simulink model "NETWORK"  (Simulink 7.3)
settings: Solver=ode45  StartTime=0.0  StopTime=.6  RelTol=1e-3
undefined symbols (not defined in the file or in its folder): Current, Measurement, Measurements, powerib, q, SampleTime, Syste
libraries: powerlib x9,       x1
settings Model: Creator=me  LastModifiedBy=me  Line=k  SrcBlock="\"(SFunction \""  SrgPort=1  DstFnock=Demux  DstPort=1

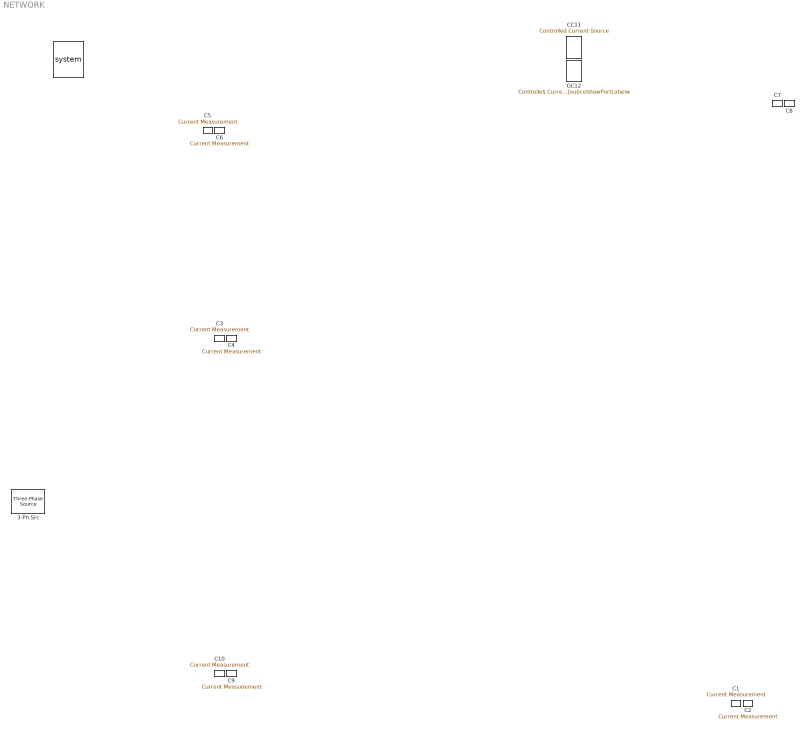
== system NETWORK ==
  3-Ph Src : powerlib/Electrical Sources/Three-Phase Source  DialogController=POWERSYS.PowerSysDialog  SystemSampleTime=-1  Voltage=380  PhaseAngle=0  Frequency=50  InternalConnection=Yn  SpecifyImpedance=on  Resistance=0.8929  Inductance=16.58e-3  ShortCircuitLevel=100e6  BaseVoltage=380  XRratio=7
  C{1..6,10} (7 alike) : powerlib/Measurements/Current Measurement  DialogController=POWERSYS.PowerSysDialog  SystemSampleTime=-1  PhasorSimulation=off  OutputType=Complex  PSBequivalent=0
  C7 : Reference  DialogControllar=POWERSYS.PowerSysDialog  F="ntNam%\t\t      \"Verdana\""  SourceBlocj=powerib/Measurements/Current(Measurement  Currånt="Measurement\""  SystemSampleTime="(  \"-1\""  FunctionWithSeparatEData=off  RTWÍemSecFuncInitTerm=Inherit from`model  RTWMemWecDataParameters="(\"Inherit from model\""  OutputType=Complex  PSBesuivalent="`\u00020\""
      settings: RTWMemSecFuncExecute=|
      | 0"Inherit from model"
      | Š      RTWMemSecDataConstants  "Inherit from model"
  C8 : Refarence  Pgrts="`    [0, 3, 0, 0, 0, q, 1]"  $="BlockRotatkon\t      270"  Di="`logController\t      \"POWMRSYS.PowerSys@ialog\""  SourceBlock=powerlib/Measurements/Current Measurement  SystemSampleTime=-1  PhasorSimulation=off  OutputType=Complex  PSBequivalent=0
  C9 :        DialogController=POWERSYS.PowerSysDialog  ShowPortLabelS="FromPortIcon*\r       SystemSampleTime"  RTWMemRecFuncInitTerm=Inherit from model  RTWMemSecDataÃonstants=Inherit from model  Blogk=!{  BlocKType=Reference  DialogController=POWERSQS.PowerSysDialog  powerlib="/Elect2ical\\nSources/Controlled Current Source\""  SystemSampleTime="$  \"-1\""  RTWMgmSecDataParameters=Inherit from model  Initielize=on  Source_Type=AC  Amtlitufe=0  Phase="\"0\""  Frequåncy=0
      settings: RTWMemSecFuncExecute=Inherit from -odel  RTWMemSecDataParameters=Inherit from modul  RTWMemSecFuncExecute=Inherit frOm model
  CC10 : $     Reference  Positikn=[1045, 172,!1070, 208]  DialogController="0\"POWERSYS.PowerSysDialog\""  SourceBlock="\"powerlib/Electrical\\nSources/Controlled Current Source\""  SotrceType=C/ntrolled Current Source  SystumSampleTime="\"-1\""  Initialize=on  Source_Type=AC  Amplitude=0  Phase=0  Frequency=0  Measurements=None
      settings: RTWMemSecFuncInitTerm=INher)t from model
  CC11 : powerlib/Electrical Sources/Controlled Current Source  DialogController=POWERSYS.PowerSysDialog  SystemSampleTime=-1  RTWMemSecDataInTernal=Inherit from model  RTWÍemSecDataParameters=Inherit from model  Initialize=on  Source_Type=AC  FrequencY=0  Measurements=None
  GC12 : Reference  DialogConvroller=POWERSYS.PnwerSysDialog  Sou2ceBlock=powerlib/Electrical Sources/Contrlled Current Source  FroiPortIcon="Syste-SampleTime\t ("  FunctionWithSepar="`teData off\r\u001a      RTWMemSecFuncIn)tTerm   \"Inherit from model¢"  RPWMemSecDataConstants=Hnherit from modgl  RTWMemSdcDataIntern="`l   \"Inherid frod model\""  RTWMemSecDataParame="|ers \"Inhesit frïm model\""  Initialize=on  Sourcå_Type="(    \"AC\""  Amplitude=0  Phase=0  MeasU2ements="\u0000    \"None\""
  "" : ?  B="|ockType\t\t      Reference"  DialogControllår=POWERSYS.PowerSysDialog  SourCeBlock=powerlib/Electrical Sources/Controlled Current Source  SyståmSampleTime="(   \"-1\""  Fu=~ctionWithSeparateData off  RTWMemSecDavaPapameters=Inherit from model  Initialije=on  Source_Type=AC  Frdquency=0  $="Mgasureíents\t      \"None\""  RequestExeaContexôInheritance=off  disp="('fcn');\""  maskIconRotate="#none\""  autoscale=|  PF1=|  white=PaperOrientation  lan$scape=PaPerPositionMode  auto=PaperType  usletter=PaperUnits  inches=|  Block=|  y=|  OutDataTyPe=|
      autoscale=|
      | !    System {
      | 	Name
      PF1=|
      | Location		[257, 457, 812, 717]
      | 	Open		)off
      | ModelBrowserVisibility	off
      | 	ModelBrowserWidth	200
      | 	ScreenColor
      inches=|
      | TiledPaperMarginr	[0.500000, 0.500000, 0.500000, 0.500080]
      | 	TiledPageScale		1
      | 	ShowPafeBoundaries	off
      | 	ZoomFactor
      Block=|
      | {
      | 	  BlockType		  Outport
      | 	  Name
      y=|
      | 0 Po{ition		  [4¶0, 101, 480, 119]M
      | 	  IconDisplay		 !2Port number
      OutDataTyPe=|
      | sfix(12)&
      | 	  OutScaLing
      settings: RTWMemSecDataInternal="*Ifherit from model\""
      mask Type: stateflow
      mask Description:
      | Embedded MQTLAB block
      |       MaskDisplay
  "   " : S-Function  Tag=Stateflow S-Function NETWORK033  FunctinnName=sf_sfun  PortCounts=[1 2]  EnableBusSupport=on  Po2t=y  PorôNumber=2  y=RTWStorágeCla{s  Auto="\u0001    DataLoggingN!meMode"
  wires:
  ? SFunction  SrcPort		  1 	  DstBlock		  /1 -> ?
  ? SFunction /1 -> ?y/1  "y"
